simulink model "kd2bd_matched_filter_clock_extraction"  (Simulink 8.0)
settings: Solver=ode45  StartTime=0.0  StopTime=100  RelTol=1e-3
undefined symbols (not defined in the file): dfilt, fdesignblkfcn, gcbh
libraries: dsparch4 x1, commrandsrc2 x1, commsource2 x1
(part 2 of 2)

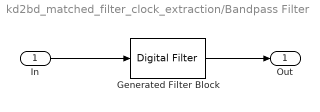
== system kd2bd_matched_filter_clock_extraction/Bandpass Filter ==
  In : Inport
  Generated Filter Block : dsparch4/Digital Filter  Tag=BlockMethodSubSystem  TypePopup=FIR (all zeros)  IIRFiltStruct=Direct form II transposed  AllPoleFiltStruct=Direct form  FIRFiltStruct=Direct form symmetric  CoeffSource=Specify via dialog  NumCoeffs=[-0.000116353334401142833 -0.000116368332113052968 -0.00011638710892303175 -0.000116409665784335083 -0.000116436003433496605 -0.000116466122390223735 -0.000116500022957299323 -0.000116537705220492747 -0.000116579169048475396 -0.000116624414092744659 -0.000116673439787554233 -0.000116726245349851838 -0.000116782829779223002 -0.000116843191857843732 -0.000116907330150437097 -0.00011697524300423972 -0.000117046928548973704 -0.000117122384696826147 -0.000117201609142434591 -0.00011728459936288125 -0.0001173713526176923 -0.000117461865948845567 -0.000117556136180784515 -0.00011765415992043934 -0.000117755933557255155 -0.000117861453263227097 -0.000117970714992942237 -0.000118083714483629054 -0.000118200447255212981 -0.000118320908610380015 -0.000118445093634646161 -0.000118572997196435238 -0.000118704613947162065 -0.000118839938321324196 -0.000118978964536599392 -0.000119121686593950951 -0.000119268098277739473 -0.000119418193155841894 -0.000119571964579777526 -0.000119729405684840815 -0.00011989050939024123 -0.000120055268399250391 -0.000120223675199355171 -0.000120395722062419935 -0.0001205714010448525 -0.000120750703987780432 -0.00012093362251723183 -0.000121120148044324201 -0.000121310271765460439 -0.000121503984662530906 -0.000121701277503122836 -0.000121902140840737347 -0.000122106565015012668 -0.000122314540151953759 -0.000122526056164170617 -0.000122741102751121409 -0.000122959669399364593 -0.000123181745382815622 -0.000123407319763013261 -0.000123636381389389979 -0.000123868918899551679 -0.000124104920719562674 -0.000124344375064238565 -0.000124587269937444608 -0.000124833593132403275 -0.000125083332232006102 -0.000125336474609134255 -0.000125593007426984715 -0.000125852917639404405 -0.000126116191991229945 -0.00012638281701863555 -0.000126652779049486264 -0.000126926064203699266 -0.000127202658393611528 -0.000127482547324353805 -0.000127765716494231764 -0.000128052151195114479 -0.000128341836512828376 -0.000128634757327559282 -0.000128930898314260083 -0.000129230243943065598 -0.000129532778479714576 -0.000129838485985977656 -0.000130147350320091999 -0.000130459355137204074 -0.000130774483889816405 -0.000131092719828243803 -0.000131414046001074368 -0.000131738445255638056 -0.000132065900238481203 -0.000132396393395848379 -0.000132729906974169863 -0.000133066423020557402 -0.000133405923383304051 -0.000133748389712393074 -0.000134093803460011581 -0.000134442145881072086 -0.000134793398033738939 -0.000135147540779963058 -0.000135504554786021941 -0.000135864420523066427 -0.000136227118267674078 -0.000136592628102409272 -0.000136960929916388484 -0.000137332003405854042 -0.000137705828074752144 -0.000138082383235319005 -0.000138461648008671666 -0.000138843601325407503 -0.000139228221926206988 -0.00013961548836244556 -0.000140005378996810808 -0.000140397872003924829 -0.000140792945370974825 -0.000141190576898348586 -0.000141590744200276305 -0.000141993424705479641 -0.000142398595657825677 -0.000142806234116987747 -0.000143216316959112052 -0.000143628820877492012 -0.000144043722383245185 -0.000144460997806000757 -0.000144880623294589426 -0.000145302574817741568 -0.000145726828164790347 -0.000146153358946381754 -0.0001465821425951894 -0.000147013154366636942 -0.000147446369339624555 -0.000147881762417263805 -0.000148319308327615447 -0.000148758981624436251 -0.000149200756687929053 -0.000149644607725500639 -0.000150090508772524186 -0.000150538433693108716 -0.000150988356180872731 -0.000151440249759725949 -0.0001518940877846534 -0.000152349843442509928 -0.00015280748975281567 -0.000153266999568560565 -0.000153728345577013107 -0.00015419150030053459 -0.000154656436097400194 -0.000155123125162624526 -0.000155591539528792744 -0.000156061651066898347 -0.000156533431487185541 -0.000157006852339997254 -0.0001574818850166287 -0.000157958500750187173 -0.000158436670616455514 -0.000158916365534763449 -0.000159397556268861572 -0.000159880213427803392 -0.000160364307466830423 -0.000160849808688264727 -0.000161336687242404222 ...(+53949 chars)]  DenCoeffs=[1 0.1]  BiQuadCoeffs=[1 0.3 0.4 1 0.1 0.2]  LatticeCoeffs=[0.2 0.4]  denIgnore=on  FiltPerSampPopup=One filter per frame  IC=0  ICnum=0  ICden=0  roundingMode=Floor  overflowMode=off  ScaleValues=1  scaleValueFracLength=14  stageInFracLength=15  stageOutFracLength=15  FilterSource=Specify via dialog  dfiltObjectName=dfilt.dffir([1 2 1])
  Out : Outport
  wires:
  In/1 -> Generated Filter Block/1
  Generated Filter Block/1 -> Out/1
